simulink model "Ilagan_Arcega_SIMULINK_LAB3_No1"  (R2024a)
settings: Solver=VariableStepAuto  StartTime=0.0  StopTime=20.0  RelTol=1e-3
settings Model: Creator=Kyla Ilagan  LastModifiedBy=Kyla Ilagan

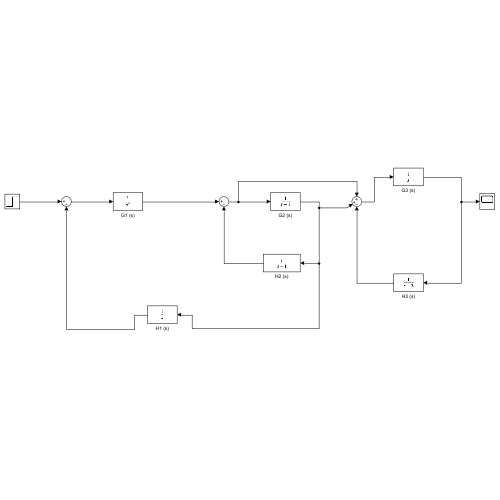
[thumbnail: Simulink's stored preview of the top-level diagram]
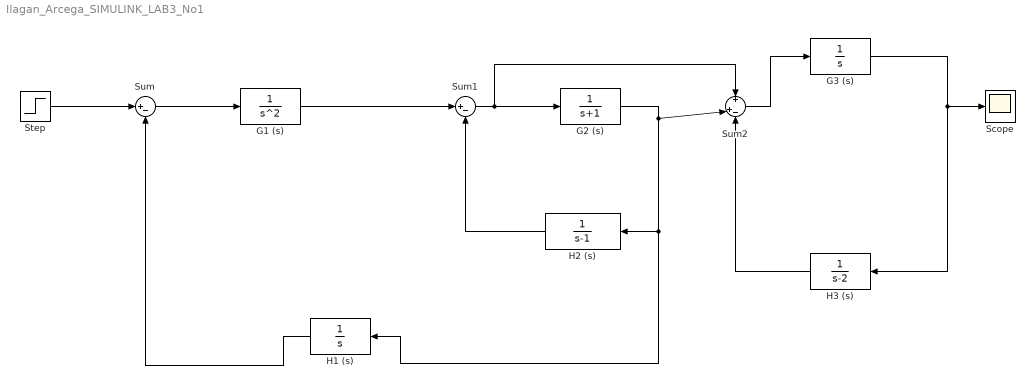
== system Ilagan_Arcega_SIMULINK_LAB3_No1 ==
  G1 (s) : TransferFcn  Numerator=[0,1]  Denominator=[1,0,0]
  G2 (s) : TransferFcn  Numerator=[0,1]  Denominator=[1,1]
  G3 (s) : TransferFcn  Numerator=[0,1]  Denominator=[1,0]
  H1 (s) : TransferFcn  Numerator=[0,1]  Denominator=[1,0]
  H2 (s) : TransferFcn  Numerator=[0,1]  Denominator=[1,-1]
  H3 (s) : TransferFcn  Numerator=[0,1]  Denominator=[1,-2]
  Scope : Scope
  Step : Step  Time=0  SampleTime=0
  Sum : Sum  Inputs=|+-
  Sum1 : Sum  Inputs=|+-
  Sum2 : Sum  Inputs=+|+-
  wires:
  H1 (s)/1 -> Sum/2
  H2 (s)/1 -> Sum1/2
  G3 (s)/1 -> H3 (s)/1, Scope/1
  Sum1/1 -> Sum2/1, G2 (s)/1
  H3 (s)/1 -> Sum2/3
  Sum2/1 -> G3 (s)/1
  G2 (s)/1 -> H1 (s)/1, H2 (s)/1, Sum2/2
  Step/1 -> Sum/1
  Sum/1 -> G1 (s)/1
  G1 (s)/1 -> Sum1/1
